simulink library "INT_EnvP_DD"  (R2016b)
settings: Solver=VariableStepAuto  StartTime=0.0  StopTime=10.0  RelTol=1e-3
settings Model: Creator=Administrator  LastModifiedBy=Administrator

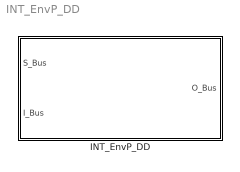
== system INT_EnvP_DD ==
  INT_EnvP_DD : Subsystem

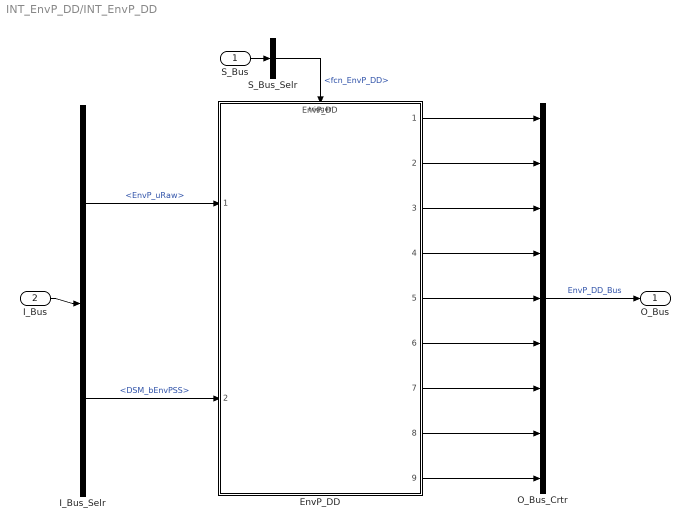
== system INT_EnvP_DD/INT_EnvP_DD ==
  S_Bus : Inport
  I_Bus : Inport  Port=2
  EnvP_DD : ModelReference  ModelNameDialog=EnvP_DD  SimulationMode=Normal  ModelReferenceVersion=1.8  TriggerPortName=function  TriggerPortTriggerType=function-call  TriggerPortStatesWhenEnabling=held
  I_Bus_Selr : BusSelector  OutputSignals=EnvP_uRaw,DSM_bEnvPSS
  O_Bus_Crtr : BusCreator  Inputs=9
  S_Bus_Selr : BusSelector  OutputSignals=fcn_EnvP_DD
  O_Bus : Outport
  wires:
  S_Bus_Selr/1 -> EnvP_DD/Trigger  "<fcn_EnvP_DD>"
  S_Bus/1 -> S_Bus_Selr/1
  I_Bus/1 -> I_Bus_Selr/1
  I_Bus_Selr/1 -> EnvP_DD/1  "<EnvP_uRaw>"
  I_Bus_Selr/2 -> EnvP_DD/2  "<DSM_bEnvPSS>"
  O_Bus_Crtr/1 -> O_Bus/1  "EnvP_DD_Bus"
  EnvP_DD/1 -> O_Bus_Crtr/1
  EnvP_DD/2 -> O_Bus_Crtr/2
  EnvP_DD/3 -> O_Bus_Crtr/3
  EnvP_DD/4 -> O_Bus_Crtr/4
  EnvP_DD/5 -> O_Bus_Crtr/5
  EnvP_DD/6 -> O_Bus_Crtr/6
  EnvP_DD/7 -> O_Bus_Crtr/7
  EnvP_DD/8 -> O_Bus_Crtr/8
  EnvP_DD/9 -> O_Bus_Crtr/9
